simulink model "Messages5"  (R2020a)
settings: Solver=VariableStepAuto  StartTime=0.0  StopTime=0.4  RelTol=1e-3
settings Model: Creator=86188  LastModifiedBy=bzhan
settings DataIOCC: ReturnWorkspaceOutputs=off
settings DebuggingCC: ArithmeticOperatorsInVariantConditions=warning
settings SFSimCC: SimUseLocalCustomCode=off  CustomCodeUndefinedFunction=UseInterfaceOnly
settings RTWCC: RTWUseLocalCustomCode=off

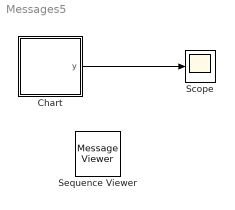
== system Messages5 ==
  Chart : Stateflow chart  TreatAsAtomicUnit=on
  Scope : Scope
  Sequence Viewer : MessageViewer
  wires:
  Chart/1(y) -> Scope/1

== stateflow chart Messages5/Chart ==
  settings: updateMethod=DISCRETE  sampleTime=0.1
  state A
    en:
    f("en_A");
    M1.data=4;
    send(M1);
    M.data=3;
    send(M);
    M1.data=3;
    send(M1);
    M1.data=2;
    send(M1);
  state B
    en:
    f("en_B");
    y=1;
  state C
    en:f("en_C");
    y=2;
  state D
    en:f("en_D");
  state E
    en:f("en_E");
  (default) -> A
  A -> B : M[M.data==3]
  B -> C : M1[M1.data==3]
  C -> D : M1[M1.data==4]
  D -> E : [M1.data==2]
  data: s function_input; M local; y output; M1 local
  function f(s):
    | function f(s)
    |   fprintf(s+"\n");
